simulink model "Sim5_MMC"  (R2021a)
settings: Solver=ode1  StartTime=0.0  StopTime=4  FixedStep=Time_Step  RelTol=1e-3
undefined symbols (not defined in the file): DiscIntNeverNeededParam, GRD00_Lg, GRD00_Rg, Time_Step, VSC01_id0
libraries: spsVoltageMeasurementLib x26, spsSeriesRLCBranchLib x24, Control_Lib x16, simulink x15, spsCurrentMeasurementLib x14, spsControlledCurrentSourceLib x12, spsControlledVoltageSourceLib x12, spsThreePhaseSourceLib x7, spsThreePhaseBreakerLib x6, spsThreePhaseVIMeasurementLib x5, spsLoadFlowBusLib x4, spsDCVoltageSourceLib x3
(part 1 of 5)
settings Model: Creator=fcolas  LastModifiedBy=fcolas
settings SolverCC: AlgebraicLoopSolver=TrustRegion
settings DebuggingCC: SFMachineParentedDataDiag=warning

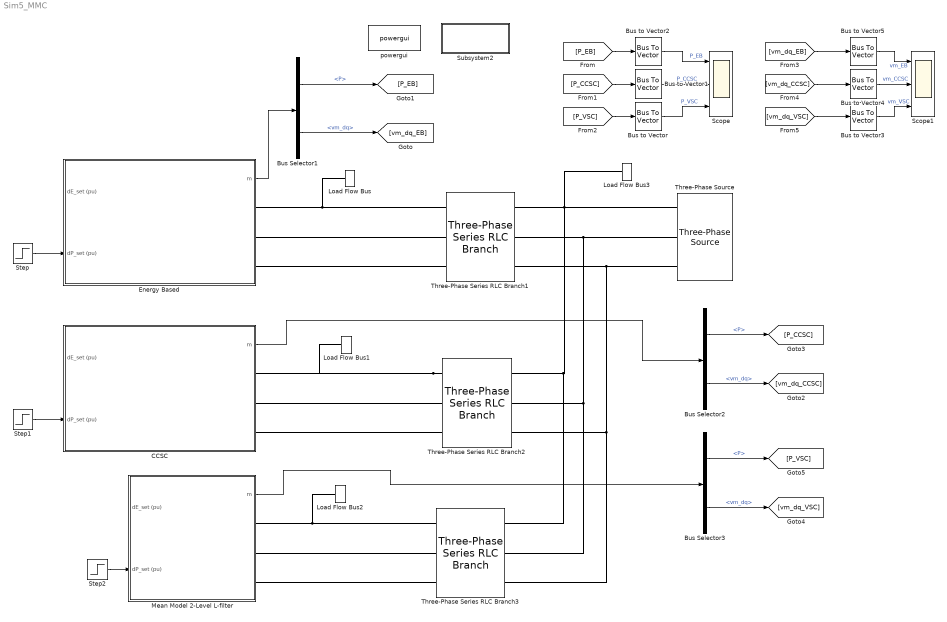
== system Sim5_MMC ==
  Bus Selector1 : BusSelector  OutputSignals=P,V.vm_dq
  Bus Selector2 : BusSelector  OutputSignals=P,V.vm_dq
  Bus Selector3 : BusSelector  OutputSignals=P,V.vm_dq
  Bus to Vector{,1..5} (6 alike) : BusToVector
  CCSC : Subsystem  mask(VSC){fn=50, Sn=1000e6, Pn=1000e6, Udcn=640e3, Time_Step=Time_Step, Un1=320e3, Un2=400e3, Rt_pu=0.005, Lt_pu=0.15, Lm_pu=500, Rm_pu=500, Larm_pu=0.18, Rarm_pu=0.005, nSM=0, Hc=40, Tr_PLL=100, Val_Freq_Support=off, R_percent=4, Rv=0.09, W_TVR=60, I_thresh_pu=1.2, DX_DR=5, Kp_Rvi_pu=0.676, I_max_pu=1.2, Tr_I_max=10, Diff_CC_fn=200, Diff_CC_zeta=1, fn_Wtot=5, zeta_Wtot=1, fn_Wdiff=3, zeta_Wdiff=1, Advanced=on, gainpopup=With Inertia, f_Inertia_Less=5, zeta_Inertia_Less=1, Param_Inertia=PI, H_GFo=5, zeta_GFo=1, LFpopup=PQ, P0=0.2, Q0=0, V0=1.0009, Theta0=0.57242}
      mask prompts: fn "Nominal Frequency (Hz)"; Sn "Nominal Apparent Power (VA)"; Pn "Nominal Power (W)"; Udcn "Nominal DC Voltage (V)"; Time_Step "Sample Time (s)"; Un1 "VSC side Nominal Ph-Ph Voltage (V)"; Un2 "Grid side Nominal Ph-Ph Voltage (V)"; Rt_pu "R (pu)"; Lt_pu "L (pu)"; Lm_pu "Rm (pu)"; Rm_pu "Lm (pu)"; Larm_pu "Arm Inductance (pu)"; Rarm_pu "Arm Resistance (pu)"; nSM "Sub-Modules number"; Hc "Hc (ms)"; Tr_PLL "Time response (ms)"; Val_Freq_Support "Frequency Support"; R_percent "Droop Gain (%)"; Rv "Damping Resistance (Rv)"; W_TVR "Dr filter"; I_thresh_pu "Current Threshold (pu)"; Kp_Rvi_pu "Kp_Rvi"; I_max_pu "I max (pu)"; Tr_I_max "Current Loop time response (ms)"; Diff_CC_fn "Bandwidth (Hz)"; Diff_CC_zeta "Damping"; fn_Wtot "Bandwidth (Hz)"; zeta_Wtot "Damping"; fn_Wdiff "Bandwidth (Hz)"; zeta_Wdiff "Damping"; gainpopup "Strategy"; f_Inertia_Less "Bandwidth (Hz)"; zeta_Inertia_Less "Damping"; H_GFo "Inertia H (s)"; zeta_GFo "Damping Ratio"; P0 "Initial Active Power (pu)"; Q0 "Initial Reactive Power (pu)"; V0 "Initial Voltage (pu)"; Theta0 "Initial Angle (°)"
      mask init:
      | % Update Name of LF bus for internal purpose
      |     %NameStr = [get_param(gcb,'Name')];% '_LF'];
      |     %set_param([gcb '/Load Flow Bus'],'ID',NameStr);    
      |     
      | % Base values
      |     fb = fn;
      |     Pb = Pn;
      |     cos_phi_n = Pn/Sn;
      |     Sb = Pb/cos_phi_n;
      |     Vn1 = Un1/sqrt(3);
      |     Vb1 = Vn1;
      |     Vn2 = Un2/sqrt(3);
      |     Vb2 = Vn2;
      |     Ib1 = Sb / 3*Vb1;
      |     Ib2 = Sb / (3*Vb2);
      |     wb = 2*pi*fb;
      |     Vdcb = Udcn;
      |     Idcb = Pb / Vdcb;
      |     Zb = (3*Vb1^2)/Sb;
      |     Lb = Zb/wb;
      |     Cb = 1/(Zb*wb);
      | 
      | % Average Model parameters
      |     Carm = 1/3*Pb/Vdcb^2*Hc/1000;
      |   
      | % PLL derivation of the parameters
      |     wn_PLL=5/Tr_PLL;
      |     zeta_PLL = 1;
      |     Kp_PLL_pu = 2*zeta_PLL*wn_PLL/wb;
      |     Ki_PLL_pu = wn_PLL^2/wb;
      |     
      | % Grid-Forming control tuning
      |     % Inertia Less
      |     wn_Inertia_Less = 2*pi*f_Inertia_Less;
      |     Ki_Inertia_Less = Lt_pu*wn_Inertia_Less^2/wb;
      |     Kp_Inertia_Less = 2*zeta_Inertia_Less*wn_Inertia_Less*Lt_pu/wb;
      |     
      |     % With Inertia
      |     Kc = 1/(Lt_pu+Larm_pu/2);
      |     kp_GFo = zeta_GFo*sqrt(2/(H_GFo*wb*Kc));
      |     kd = 2*H_GFo*kp_GFo*Kc*wb;
      |     
      | % Set the chosen strategy
      |     if (gainpopup == 1)
      |         Chosen_Strategy = 1;
      |     elseif (gainpopup == 2)
      |         if (Param_Inertia == 1)
      |             Chosen_Strategy = 2;
      |         elseif (Param_Inertia == 2)
      |             Chosen_Strategy = 3;
      |         end
      |     end
      | 
      | % Differential Current controller (CCSC)
      | 
      |     HL = 1/2*Larm_pu*Lb*Idcb^2/Pb; 
      |     Diff_CC_wn = 2*pi*Diff_CC_fn;
      |     Diff_CC_ki= 2*HL*Diff_CC_wn*Diff_CC_wn;
      |     Diff_CC_kp= (4*Diff_CC_zeta*Diff_CC_wn*HL)-(Rarm_pu);
      | 
      | %% Energy Sum W tot Per phase control design
      |     Hc_W    = 0.5*Carm*(Udcn^2)/Pn;    
      |     wn_Wtot     = 2*pi*fn_Wtot;
      |     Kp_Wtot_pu  = 2*zeta_Wtot*wn_Wtot*2*Hc_W;
      |     Ki_Wtot_pu  = wn_Wtot*wn_Wtot*2*Hc_W;
      | 
      | %% Control difference (balancing)  W diff Per phase control design  
      |     wn_Wdiff    = 2*pi*fn_Wdiff;
      |     Kp_Wdiff_pu = 2*zeta_Wdiff*wn_Wdiff*2*Hc_W;
      |     Ki_Wdiff_pu = wn_Wdiff*wn_Wdiff*2*Hc_W;
      |     
      | % Set the frequency droop gain
      |     R = R_percent / 100;
      | 
      | % Compute the delay compensation between control and power parts
      |     if (Time_Step == -1)
      |         Solver_Time_Step = 0;
      |     else
      |         Solver_Time_Step = Time_Step;
      |     end
      | 
      | % Compute Initial Voltage of VSC 
      | %   from steady-state output transformer model and Loadflow result
      |     
      |     %Initialize correctly the LoadFlow bus parameters connected to PCC
      |     VLF = V0;
      |     ThetaLF = Theta0;
      |     %if (LFpopup == 'PQ')
      |     %    VLF = 1;
      |     %    ThetaLF = 0;
      |     %elseif (LFpopup == 'PV')
      |     %%    VLF = V0;
      |     %    ThetaLF = 0;        
      |     %end
      |     %set_param([gcb '/Load Flow Bus'],'Vref',num2str(VLF),'Vangle',num2str(ThetaLF));
      |     
      |     R1_pu = Rt_pu/2+Rarm_pu/2;
      |     L1_pu = Lt_pu/2+Larm_pu/2;
      |     R2_pu = Rt_pu/2;
      |     L2_pu = Lt_pu/2;
      |     X1_pu = L1_pu;
      |     X2_pu = L2_pu;
      |     Xm_pu = Lm_pu;
      |     
      |     Zm_pu = 1/(1/Rm_pu+1/(1i*Xm_pu));
      | 
      |     S0=P0+1i*Q0;
      |     I2 = conj(S0)/(V0);
      | 
      |     Vm = (R2_pu+1i*X2_pu)*I2 + V0;
      |     Im = Vm/Zm_pu;
      | 
      |     I1 = I2 + Im;
      |     V1 = (R1_pu+1i*X1_pu) * I1 + Vm;
      | 
      |     Vvsc0 = abs(V1);
      |     Theta_vsc0 = angle(V1) * 180/pi+Theta0;
      |     
      |     Va0 = Vvsc0*sqrt(2)*Vb1*sin(Theta_vsc0*pi/180);
      |     Vb0 = Vvsc0*sqrt(2)*Vb1*sin(Theta_vsc0*pi/180-2*pi/3);
      |     Vc0 = Vvsc0*sqrt(2)*Vb1*sin(Theta_vsc0*pi/180+2*pi/3);
      |     
      | % Generate string to display LF results on Mask
      |     %str_tmp = fprintf("Vvsc0 = %d, Theta_vsc0 = %d°",Vvsc0,Theta_vsc0);
      |     mo = get_param(gcb,'MaskObject');
      |     mo.getDialogControl('LF_vsc_str').Prompt = ['V0 = ', num2str(Vvsc0),' pu, Angle = ', num2str(Theta_vsc0),'°'];
      |     mo.getDialogControl('LF_pcc_str').Prompt = ['V0 = ', num2str(V0),' pu, Angle = ', num2str(Theta0),'°'];
      |     mo.getDialogControl('LF_pcc_Power_str').Prompt = ['P0 = ', num2str(P0),' pu, Q0 = ', num2str(Q0),' pu'];
      |     %set_param([gcb],'LF_str',str_tmp);
      settings: OpenFcn=|
      | NameStr = get_param(gcb,'Name');
      | open_system(gcbh, 'Mask');
      | 
      | h2AllOpenDlgs = DAStudio.ToolRoot.getOpenDialogs;
      | 
      | for i=1:length(h2AllOpenDlgs)
      |     try
      |          %disp(h2AllOpenDlgs(i).getSource.getBlock.Name);
      |         Dialog_block_name = h2AllOpenDlgs(i).getSource.getBlock.Name;
      |          %strcmp(Dialog_block_name, NameStr),
      |         if (strcmp(h2AllOpenDlgs(i).getSource.getBlock.Name, NameStr))
      |             iPos = h2AllOpenDlgs(i).position;
      |             h2AllOpenDlgs(i).position = [iPos(1)   iPos(2)   iPos(3)*1.4   iPos(4)];
      |         end
      |     end
      | end
      mask Callback Advanced:
      | % Get the mask parameter values. This is a cell
      | %   array of character vectors.
      | maskStr = get_param(gcb,'Advanced');
      | p=Simulink.Mask.get(gcb);
      | 
      | % The pop-up menu is the first mask parameter.
      | %   Check the value selected in the pop-up
      | if strcmp(maskStr,'on'),
      | 
      |     % Set the visibility of both parameters on when
      |     %   User-defined is selected in the pop-up.
      |     p.getDialogControl('TVR').Visible='on';
      |     p.getDialogControl('TVI').Visible='on';
      |     %p.getDialogControl('LC_Filter').Visible='on';
      |     p.getDialogControl('Current_Sat').Visible='on';
      |     p.getDialogControl('MMC_Control').Visible='on';
      |     %p.getDialogControl('Param_Strat_3').Visible='off';
      | 
      | 
      | else
      | 
      |     % Set the visibility of both parameters on when
      |     %   User-defined is selected in the pop-up.
      |     p.getDialogControl('TVR').Visible='off';
      |     p.getDialogControl('TVI').Visible='off';
      |     %p.getDialogControl('LC_Filter').Visible='off';
      |     p.getDialogControl('Current_Sat').Visible='off';
      |     p.getDialogControl('MMC_Control').Visible='off';
      |     %p.getDialogControl('Param_Strat_3').Visible='off';
      | 
      | end
      mask TypeOptions gainpopup: Inertia Less | With Inertia
      mask Callback gainpopup:
      | % Get the mask parameter values. This is a cell
      | %   array of character vectors.
      | maskStr = get_param(gcb,'gainpopup');
      | p=Simulink.Mask.get(gcb);
      | 
      | % The pop-up menu is the first mask parameter.
      | %   Check the value selected in the pop-up
      | if strcmp(maskStr,'Inertia Less'),
      | 
      |     % Set the visibility of both parameters on when
      |     %   User-defined is selected in the pop-up.
      |     p.getDialogControl('No_Inertia').Visible='on';
      |     p.getDialogControl('Inertia').Visible='off';
      |     %p.getDialogControl('Param_Strat_3').Visible='off';
      | 
      | 
      | elseif strcmp(maskStr,'With Inertia'),
      | 
      |     % Set the visibility of both parameters on when
      |     %   User-defined is selected in the pop-up.
      |     p.getDialogControl('No_Inertia').Visible='off';
      |     p.getDialogControl('Inertia').Visible='on';
      |     %p.getDialogControl('Param_Strat_3').Visible='off';
      | 
      | 
      |     % Turn off the visibility of the Value field
      |     %   when User-defined is not selected.
      | 
      | else
      | 
      |     % Set the visibility of both parameters on when
      |     %   User-defined is selected in the pop-up.
      |     p.getDialogControl('No_Inertia').Visible='off';
      |     p.getDialogControl('Inertia').Visible='off';
      |     %p.getDialogControl('Param_Strat_3').Visible='off';
      | 
      | end
      mask TypeOptions Param_Inertia: VSM | PI
      mask TypeOptions LFpopup: Swing | PQ | PV
      mask Callback LFpopup:
      | % Get the mask parameter values. This is a cell
      | %   array of character vectors.
      | maskStr = get_param(gcb,'LFpopup');
      | p=Simulink.Mask.get(gcb);
      | 
      | % The pop-up menu is the first mask parameter.
      | %   Check the value selected in the pop-up
      | if strcmp(maskStr,'Swing'),
      | 
      |     % Set the visibility of both parameters on when
      |     %   User-defined is selected in the pop-up.
      |     p.getParameter('P0').Visible='off';
      |     p.getParameter('Q0').Visible='off';
      |     p.getParameter('V0').Visible='on';
      |     p.getParameter('Theta0').Visible='on';
      |     set_param([gcb '/Source_For_LF'],'BusType','swing');
      | 
      | elseif strcmp(maskStr,'PQ'),
      | 
      |     % Set the visibility of both parameters on when
      |     %   User-defined is selected in the pop-up.
      |     p.getParameter('P0').Visible='on';
      |     p.getParameter('Q0').Visible='on';
      |     p.getParameter('V0').Visible='off';
      |     p.getParameter('Theta0').Visible='off';
      |     set_param([gcb '/Source_For_LF'],'BusType','PQ');
      | 
      |     % Turn off the visibility of the Value field
      |     %   when User-defined is not selected.
      | else
      | 
      |     % Set the visibility of both parameters on when
      |     %   User-defined is selected in the pop-up.
      |     p.getParameter('P0').Visible='on';
      |     p.getParameter('Q0').Visible='off';
      |     p.getParameter('V0').Visible='on';
      |     p.getParameter('Theta0').Visible='off';
      |     set_param([gcb '/Source_For_LF'],'BusType','PV');
      | 
      | end
      mask DialogControl Nominal_Param Prompt: Nominal Value
      mask DialogControl Container20 Prompt: Passive Components
      mask DialogControl Container21 Prompt: Output Transformer
      mask DialogControl Container22 Prompt: Sub-Modules & Arm
      mask DialogControl Control_Param Prompt: Control Parameter
      mask DialogControl Container13 Prompt: PLL
      mask DialogControl Container14 Prompt: Frequency Support
      mask DialogControl TVR Prompt: Transient Virtual Resistor
      mask DialogControl TVI Prompt: Virtual Impedance
      mask DialogControl Current_Sat Prompt: Current Limitation
      mask DialogControl MMC_Control Prompt: MMC Controller
      mask DialogControl Container27 Prompt: Differential Current Controller
      mask DialogControl Container26 Prompt: Wtot Controller
      mask DialogControl Container28 Prompt: Wdiff Controller
      mask DialogControl Container18 Prompt: Control Strategy
      mask DialogControl LF_Param Prompt: Loadflow
      mask DialogControl Control4 Prompt: Initial Operating Point
      mask DialogControl Container24 Prompt: VSC side
      mask DialogControl LF_vsc_str Prompt: V0 = 1.0039 pu, Angle = 3.3291°
      mask DialogControl Container25 Prompt: PCC
      mask DialogControl LF_pcc_str Prompt: V0 = 1.0009 pu, Angle = 0.57242°
      mask DialogControl LF_pcc_Power_str Prompt: P0 = 0.2 pu, Q0 = 0 pu
      mask DialogControl UpdateLoadflow Prompt: Update Loadflow
      mask DialogControl UpdateLoadflow Callback: LoadFlow_VSC
      mask Display:
      | % Q1
      | x1=-0.07;
      | y1=+0.03;
      | plot([0.4 0.4]+x1,[0.90,0.80]+y1)
      | plot([0.4 0.33]+x1,[0.80 0.74]+y1)
      | plot([0.33 0.33]+x1,[0.78 0.66]+y1)
      | plot([0.33 0.4]+x1,[0.70 0.64]+y1)
      | plot([0.4 0.4]+x1,[0.64 0.55]+y1)
      | plot([0.38 0.40 0.35]+x1,[0.68 0.64 0.64]+y1)
      | plot([0.30 0.30]+x1,[0.74 0.7]+y1)
      | plot([0.29 0.27]+x1,[0.72 0.72]+y1)
      | % Q2
      | y1=y1-0.51;
      | plot([0.4 0.4]+x1,[0.90,0.80]+y1)
      | plot([0.4 0.33]+x1,[0.80 0.74]+y1)
      | plot([0.33 0.33]+x1,[0.78 0.66]+y1)
      | plot([0.33 0.4]+x1,[0.70 0.64]+y1)
      | plot([0.4 0.4]+x1,[0.64 0.55]+y1)
      | plot([0.39 0.40 0.35]+x1,[0.68 0.64 0.64]+y1)
      | plot([0.30 0.30]+x1,[0.75 0.7]+y1)
      | plot([0.29 0.27]+x1,[0.72 0.72]+y1)
      | % Q3
      | y1=y1+0.51;
      | x1=x1+0.22+0.1;
      | plot([0.4 0.4]+x1,[0.90,0.80]+y1)
      | plot([0.4 0.33]+x1,[0.80 0.74]+y1)
      | plot([0.33 0.33]+x1,[0.78 0.66]+y1)
      | plot([0.33 0.4]+x1,[0.70 0.64]+y1)
      | plot([0.4 0.4]+x1,[0.64 0.55]+y1)
      | plot([0.39 0.41 0.34]+x1,[0.68 0.64 0.64]+y1)
      | plot([0.30 0.30]+x1,[0.75 0.7]+y1)
      | plot([0.29 0.27]+x1,[0.72 0.72]+y1)
      | % Q4
      | y1=y1-0.51;
      | x1=x1;
      | plot([0.4 0.4]+x1,[0.90,0.80]+y1)
      | plot([0.4 0.33]+x1,[0.80 0.74]+y1)
      | plot([0.33 0.33]+x1,[0.78 0.66]+y1)
      | plot([0.33 0.4]+x1,[0.70 0.64]+y1)
      | plot([0.4 0.4]+x1,[0.64 0.55]+y1)
      | plot([0.39 0.41 0.34]+x1,[0.68 0.64 0.64]+y1)
      | plot([0.30 0.30]+x1,[0.75 0.7]+y1)
      | plot([0.29 0.26]+x1,[0.72 0.72]+y1)
      | %
      | x1=-0.05;
      | y1=+0.03;
      | plot([0.90 0.40]+x1,[0.9 0.9]+y1)
      | plot([0.90 0.40]+x1,[0.04 0.04]+y1)
      | %
      | 
      | plot([0.69 0.42]+x1,[0.4 0.4]+y1)
      | plot([0.38 0.22]+x1,[0.52 0.52]+y1)
      | plot([0.22 0.22]+x1,[0.52 0.54]+y1)
      | plot([0.22 0.22]+x1,[0.56 0.58]+y1)
      | plot([0.22 0.22]+x1,[0.60 0.63]+y1)
      | %
      | plot([0.35 0.22]+x1,[0.4 0.4]+y1)
      | plot([0.22 0.22]+x1,[0.4 0.37]+y1)
      | plot([0.22 0.22]+x1,[0.4 0.37]+y1)
      | plot([0.22 0.22]+x1,[0.35 0.32]+y1)
      | plot([0.22 0.22]+x1,[0.30 0.27]+y1)
      | %
      | plot([0.38 0.38]+x1,[ 0.55 0.38]+y1)
      | plot([0.7 0.7]+x1,[0.55 0.3]+y1)
      | %
      | % D1
      | x1=-0.07;
      | y1=+0.03;
      | plot([0.4 0.45]+x1,[0.84,0.84]+y1)
      | plot([0.45 0.45]+x1,[0.84,0.75]+y1)
      | plot([0.45 0.41]+x1,[0.75,0.72]+y1)
      | plot([0.45 0.48]+x1,[0.75,0.72]+y1)
      | plot([0.41 0.48]+x1,[0.72,0.72]+y1)
      | plot([0.45 0.45]+x1,[0.72,0.6]+y1)
      | plot([0.4 0.45]+x1,[0.6,0.6]+y1)
      | % D2
      | x1=x1+0.22+0.1;
      | plot([0.4 0.45]+x1,[0.84,0.84]+y1)
      | plot([0.45 0.45]+x1,[0.84,0.75]+y1)
      | plot([0.45 0.43]+x1,[0.75,0.72]+y1)
      | plot([0.45 0.48]+x1,[0.75,0.72]+y1)
      | %
      | plot([0.43 0.48]+x1,[0.72,0.72]+y1)
      | plot([0.45 0.45]+x1,[0.72,0.6]+y1)
      | plot([0.4 0.45]+x1,[0.6,0.6]+y1)
      | % D3
      | x1=x1-0.22-0.1;
      | y1=y1-0.5;
      | plot([0.4 0.45]+x1,[0.84,0.84]+y1)
      | plot([0.45 0.45]+x1,[0.84,0.75]+y1)
      | plot([0.45 0.41]+x1,[0.75,0.72]+y1)
      | plot([0.45 0.48]+x1,[0.75,0.72]+y1)
      | plot([0.41 0.48]+x1,[0.72,0.72]+y1)
      | plot([0.45 0.45]+x1,[0.72,0.6]+y1)
      | plot([0.4 0.45]+x1,[0.6,0.6]+y1)
      | % D4
      | x1=x1+0.22+0.1;
      | plot([0.4 0.45]+x1,[0.84,0.84]+y1)
      | plot([0.45 0.45]+x1,[0.84,0.75]+y1)
      | plot([0.45 0.43]+x1,[0.75,0.72]+y1)
      | plot([0.45 0.48]+x1,[0.75,0.72]+y1)
      | plot([0.43 0.48]+x1,[0.72,0.72]+y1)
      | plot([0.45 0.45]+x1,[0.72,0.6]+y1)
      | plot([0.40 0.45]+x1,[0.6,0.6]+y1)
      | disp('MMC GFo');
      | port_label('input',1,'dE_set (pu)');
      | port_label('input',2,'dP_set (pu)');
      | port_label('output',1,'m');
      | port_label('rconn',1,'A');
      | port_label('rconn',2,'B');
      | port_label('rconn',3,'C');
  Energy Based : Subsystem  mask(VSC){fn=50, Sn=1000e6, Pn=1000e6, Udcn=640e3, Time_Step=Time_Step, Un1=320e3, Un2=400e3, Rt_pu=0.005, Lt_pu=0.15, Lm_pu=500, Rm_pu=500, Larm_pu=0.18, Rarm_pu=0.005, nSM=0, Hc=40, Tr_PLL=100, Val_Freq_Support=off, R_percent=4, Rv=0.09, W_TVR=60, I_thresh_pu=1.2, DX_DR=5, Kp_Rvi_pu=0.676, I_max_pu=1.2, Tr_I_max=10, Diff_CC_fn=200, Diff_CC_zeta=1, fn_Wtot=5, zeta_Wtot=1, fn_Wdiff=3, zeta_Wdiff=1, Advanced=on, gainpopup=With Inertia, f_Inertia_Less=5, zeta_Inertia_Less=1, Param_Inertia=PI, H_GFo=5, zeta_GFo=0.7, LFpopup=PQ, P0=0.2, Q0=0, V0=1.0009, Theta0=0.57242}
      mask prompts: fn "Nominal Frequency (Hz)"; Sn "Nominal Apparent Power (VA)"; Pn "Nominal Power (W)"; Udcn "Nominal DC Voltage (V)"; Time_Step "Sample Time (s)"; Un1 "VSC side Nominal Ph-Ph Voltage (V)"; Un2 "Grid side Nominal Ph-Ph Voltage (V)"; Rt_pu "R (pu)"; Lt_pu "L (pu)"; Lm_pu "Rm (pu)"; Rm_pu "Lm (pu)"; Larm_pu "Arm Inductance (pu)"; Rarm_pu "Arm Resistance (pu)"; nSM "Sub-Modules number"; Hc "Hc (ms)"; Tr_PLL "Time response (ms)"; Val_Freq_Support "Frequency Support"; R_percent "Droop Gain (%)"; Rv "Damping Resistance (Rv)"; W_TVR "Dr filter"; I_thresh_pu "Current Threshold (pu)"; Kp_Rvi_pu "Kp_Rvi"; I_max_pu "I max (pu)"; Tr_I_max "Current Loop time response (ms)"; Diff_CC_fn "Bandwidth (Hz)"; Diff_CC_zeta "Damping"; fn_Wtot "Bandwidth (Hz)"; zeta_Wtot "Damping"; fn_Wdiff "Bandwidth (Hz)"; zeta_Wdiff "Damping"; gainpopup "Strategy"; f_Inertia_Less "Bandwidth (Hz)"; zeta_Inertia_Less "Damping"; H_GFo "Inertia H (s)"; zeta_GFo "Damping Ratio"; P0 "Initial Active Power (pu)"; Q0 "Initial Reactive Power (pu)"; V0 "Initial Voltage (pu)"; Theta0 "Initial Angle (°)"
      mask init: same as Sim5_MMC/CCSC
      settings: OpenFcn=|
      | NameStr = get_param(gcb,'Name');
      | open_system(gcbh, 'Mask');
      | 
      | h2AllOpenDlgs = DAStudio.ToolRoot.getOpenDialogs;
      | 
      | for i=1:length(h2AllOpenDlgs)
      |     try
      |          %disp(h2AllOpenDlgs(i).getSource.getBlock.Name);
      |         Dialog_block_name = h2AllOpenDlgs(i).getSource.getBlock.Name;
      |          %strcmp(Dialog_block_name, NameStr),
      |         if (strcmp(h2AllOpenDlgs(i).getSource.getBlock.Name, NameStr))
      |             iPos = h2AllOpenDlgs(i).position;
      |             h2AllOpenDlgs(i).position = [iPos(1)   iPos(2)   iPos(3)*1.4   iPos(4)];
      |         end
      |     end
      | end
      mask Callback Advanced:
      | % Get the mask parameter values. This is a cell
      | %   array of character vectors.
      | maskStr = get_param(gcb,'Advanced');
      | p=Simulink.Mask.get(gcb);
      | 
      | % The pop-up menu is the first mask parameter.
      | %   Check the value selected in the pop-up
      | if strcmp(maskStr,'on'),
      | 
      |     % Set the visibility of both parameters on when
      |     %   User-defined is selected in the pop-up.
      |     p.getDialogControl('TVR').Visible='on';
      |     p.getDialogControl('TVI').Visible='on';
      |     %p.getDialogControl('LC_Filter').Visible='on';
      |     p.getDialogControl('Current_Sat').Visible='on';
      |     p.getDialogControl('MMC_Control').Visible='on';
      |     %p.getDialogControl('Param_Strat_3').Visible='off';
      | 
      | 
      | else
      | 
      |     % Set the visibility of both parameters on when
      |     %   User-defined is selected in the pop-up.
      |     p.getDialogControl('TVR').Visible='off';
      |     p.getDialogControl('TVI').Visible='off';
      |     %p.getDialogControl('LC_Filter').Visible='off';
      |     p.getDialogControl('Current_Sat').Visible='off';
      |     p.getDialogControl('MMC_Control').Visible='off';
      |     %p.getDialogControl('Param_Strat_3').Visible='off';
      | 
      | end
      mask TypeOptions gainpopup: Inertia Less | With Inertia
      mask Callback gainpopup:
      | % Get the mask parameter values. This is a cell
      | %   array of character vectors.
      | maskStr = get_param(gcb,'gainpopup');
      | p=Simulink.Mask.get(gcb);
      | 
      | % The pop-up menu is the first mask parameter.
      | %   Check the value selected in the pop-up
      | if strcmp(maskStr,'Inertia Less'),
      | 
      |     % Set the visibility of both parameters on when
      |     %   User-defined is selected in the pop-up.
      |     p.getDialogControl('No_Inertia').Visible='on';
      |     p.getDialogControl('Inertia').Visible='off';
      |     %p.getDialogControl('Param_Strat_3').Visible='off';
      | 
      | 
      | elseif strcmp(maskStr,'With Inertia'),
      | 
      |     % Set the visibility of both parameters on when
      |     %   User-defined is selected in the pop-up.
      |     p.getDialogControl('No_Inertia').Visible='off';
      |     p.getDialogControl('Inertia').Visible='on';
      |     %p.getDialogControl('Param_Strat_3').Visible='off';
      | 
      | 
      |     % Turn off the visibility of the Value field
      |     %   when User-defined is not selected.
      | 
      | else
      | 
      |     % Set the visibility of both parameters on when
      |     %   User-defined is selected in the pop-up.
      |     p.getDialogControl('No_Inertia').Visible='off';
      |     p.getDialogControl('Inertia').Visible='off';
      |     %p.getDialogControl('Param_Strat_3').Visible='off';
      | 
      | end
      mask TypeOptions Param_Inertia: VSM | PI
      mask TypeOptions LFpopup: Swing | PQ | PV
      mask Callback LFpopup:
      | % Get the mask parameter values. This is a cell
      | %   array of character vectors.
      | maskStr = get_param(gcb,'LFpopup');
      | p=Simulink.Mask.get(gcb);
      | 
      | % The pop-up menu is the first mask parameter.
      | %   Check the value selected in the pop-up
      | if strcmp(maskStr,'Swing'),
      | 
      |     % Set the visibility of both parameters on when
      |     %   User-defined is selected in the pop-up.
      |     p.getParameter('P0').Visible='off';
      |     p.getParameter('Q0').Visible='off';
      |     p.getParameter('V0').Visible='on';
      |     p.getParameter('Theta0').Visible='on';
      |     set_param([gcb '/Source_For_LF'],'BusType','swing');
      | 
      | elseif strcmp(maskStr,'PQ'),
      | 
      |     % Set the visibility of both parameters on when
      |     %   User-defined is selected in the pop-up.
      |     p.getParameter('P0').Visible='on';
      |     p.getParameter('Q0').Visible='on';
      |     p.getParameter('V0').Visible='off';
      |     p.getParameter('Theta0').Visible='off';
      |     set_param([gcb '/Source_For_LF'],'BusType','PQ');
      | 
      |     % Turn off the visibility of the Value field
      |     %   when User-defined is not selected.
      | else
      | 
      |     % Set the visibility of both parameters on when
      |     %   User-defined is selected in the pop-up.
      |     p.getParameter('P0').Visible='on';
      |     p.getParameter('Q0').Visible='off';
      |     p.getParameter('V0').Visible='on';
      |     p.getParameter('Theta0').Visible='off';
      |     set_param([gcb '/Source_For_LF'],'BusType','PV');
      | 
      | end
      mask DialogControl Nominal_Param Prompt: Nominal Value
      mask DialogControl Container20 Prompt: Passive Components
      mask DialogControl Container21 Prompt: Output Transformer
      mask DialogControl Container22 Prompt: Sub-Modules & Arm
      mask DialogControl Control_Param Prompt: Control Parameter
      mask DialogControl Container13 Prompt: PLL
      mask DialogControl Container14 Prompt: Frequency Support
      mask DialogControl TVR Prompt: Transient Virtual Resistor
      mask DialogControl TVI Prompt: Virtual Impedance
      mask DialogControl Current_Sat Prompt: Current Limitation
      mask DialogControl MMC_Control Prompt: MMC Controller
      mask DialogControl Container27 Prompt: Differential Current Controller
      mask DialogControl Container26 Prompt: Wtot Controller
      mask DialogControl Container28 Prompt: Wdiff Controller
      mask DialogControl Container18 Prompt: Control Strategy
      mask DialogControl LF_Param Prompt: Loadflow
      mask DialogControl Control4 Prompt: Initial Operating Point
      mask DialogControl Container24 Prompt: VSC side
      mask DialogControl LF_vsc_str Prompt: V0 = 1.0039 pu, Angle = 3.3291°
      mask DialogControl Container25 Prompt: PCC
      mask DialogControl LF_pcc_str Prompt: V0 = 1.0009 pu, Angle = 0.57242°
      mask DialogControl LF_pcc_Power_str Prompt: P0 = 0.2 pu, Q0 = 0 pu
      mask DialogControl UpdateLoadflow Prompt: Update Loadflow
      mask DialogControl UpdateLoadflow Callback: LoadFlow_VSC
      mask Display:
      | % Q1
      | x1=-0.07;
      | y1=+0.03;
      | plot([0.4 0.4]+x1,[0.90,0.80]+y1)
      | plot([0.4 0.33]+x1,[0.80 0.74]+y1)
      | plot([0.33 0.33]+x1,[0.78 0.66]+y1)
      | plot([0.33 0.4]+x1,[0.70 0.64]+y1)
      | plot([0.4 0.4]+x1,[0.64 0.55]+y1)
      | plot([0.38 0.40 0.35]+x1,[0.68 0.64 0.64]+y1)
      | plot([0.30 0.30]+x1,[0.74 0.7]+y1)
      | plot([0.29 0.27]+x1,[0.72 0.72]+y1)
      | % Q2
      | y1=y1-0.51;
      | plot([0.4 0.4]+x1,[0.90,0.80]+y1)
      | plot([0.4 0.33]+x1,[0.80 0.74]+y1)
      | plot([0.33 0.33]+x1,[0.78 0.66]+y1)
      | plot([0.33 0.4]+x1,[0.70 0.64]+y1)
      | plot([0.4 0.4]+x1,[0.64 0.55]+y1)
      | plot([0.39 0.40 0.35]+x1,[0.68 0.64 0.64]+y1)
      | plot([0.30 0.30]+x1,[0.75 0.7]+y1)
      | plot([0.29 0.27]+x1,[0.72 0.72]+y1)
      | % Q3
      | y1=y1+0.51;
      | x1=x1+0.22+0.1;
      | plot([0.4 0.4]+x1,[0.90,0.80]+y1)
      | plot([0.4 0.33]+x1,[0.80 0.74]+y1)
      | plot([0.33 0.33]+x1,[0.78 0.66]+y1)
      | plot([0.33 0.4]+x1,[0.70 0.64]+y1)
      | plot([0.4 0.4]+x1,[0.64 0.55]+y1)
      | plot([0.39 0.41 0.34]+x1,[0.68 0.64 0.64]+y1)
      | plot([0.30 0.30]+x1,[0.75 0.7]+y1)
      | plot([0.29 0.27]+x1,[0.72 0.72]+y1)
      | % Q4
      | y1=y1-0.51;
      | x1=x1;
      | plot([0.4 0.4]+x1,[0.90,0.80]+y1)
      | plot([0.4 0.33]+x1,[0.80 0.74]+y1)
      | plot([0.33 0.33]+x1,[0.78 0.66]+y1)
      | plot([0.33 0.4]+x1,[0.70 0.64]+y1)
      | plot([0.4 0.4]+x1,[0.64 0.55]+y1)
      | plot([0.39 0.41 0.34]+x1,[0.68 0.64 0.64]+y1)
      | plot([0.30 0.30]+x1,[0.75 0.7]+y1)
      | plot([0.29 0.26]+x1,[0.72 0.72]+y1)
      | %
      | x1=-0.05;
      | y1=+0.03;
      | plot([0.90 0.40]+x1,[0.9 0.9]+y1)
      | plot([0.90 0.40]+x1,[0.04 0.04]+y1)
      | %
      | 
      | plot([0.69 0.42]+x1,[0.4 0.4]+y1)
      | plot([0.38 0.22]+x1,[0.52 0.52]+y1)
      | plot([0.22 0.22]+x1,[0.52 0.54]+y1)
      | plot([0.22 0.22]+x1,[0.56 0.58]+y1)
      | plot([0.22 0.22]+x1,[0.60 0.63]+y1)
      | %
      | plot([0.35 0.22]+x1,[0.4 0.4]+y1)
      | plot([0.22 0.22]+x1,[0.4 0.37]+y1)
      | plot([0.22 0.22]+x1,[0.4 0.37]+y1)
      | plot([0.22 0.22]+x1,[0.35 0.32]+y1)
      | plot([0.22 0.22]+x1,[0.30 0.27]+y1)
      | %
      | plot([0.38 0.38]+x1,[ 0.55 0.38]+y1)
      | plot([0.7 0.7]+x1,[0.55 0.3]+y1)
      | %
      | % D1
      | x1=-0.07;
      | y1=+0.03;
      | plot([0.4 0.45]+x1,[0.84,0.84]+y1)
      | plot([0.45 0.45]+x1,[0.84,0.75]+y1)
      | plot([0.45 0.41]+x1,[0.75,0.72]+y1)
      | plot([0.45 0.48]+x1,[0.75,0.72]+y1)
      | plot([0.41 0.48]+x1,[0.72,0.72]+y1)
      | plot([0.45 0.45]+x1,[0.72,0.6]+y1)
      | plot([0.4 0.45]+x1,[0.6,0.6]+y1)
      | % D2
      | x1=x1+0.22+0.1;
      | plot([0.4 0.45]+x1,[0.84,0.84]+y1)
      | plot([0.45 0.45]+x1,[0.84,0.75]+y1)
      | plot([0.45 0.43]+x1,[0.75,0.72]+y1)
      | plot([0.45 0.48]+x1,[0.75,0.72]+y1)
      | %
      | plot([0.43 0.48]+x1,[0.72,0.72]+y1)
      | plot([0.45 0.45]+x1,[0.72,0.6]+y1)
      | plot([0.4 0.45]+x1,[0.6,0.6]+y1)
      | % D3
      | x1=x1-0.22-0.1;
      | y1=y1-0.5;
      | plot([0.4 0.45]+x1,[0.84,0.84]+y1)
      | plot([0.45 0.45]+x1,[0.84,0.75]+y1)
      | plot([0.45 0.41]+x1,[0.75,0.72]+y1)
      | plot([0.45 0.48]+x1,[0.75,0.72]+y1)
      | plot([0.41 0.48]+x1,[0.72,0.72]+y1)
      | plot([0.45 0.45]+x1,[0.72,0.6]+y1)
      | plot([0.4 0.45]+x1,[0.6,0.6]+y1)
      | % D4
      | x1=x1+0.22+0.1;
      | plot([0.4 0.45]+x1,[0.84,0.84]+y1)
      | plot([0.45 0.45]+x1,[0.84,0.75]+y1)
      | plot([0.45 0.43]+x1,[0.75,0.72]+y1)
      | plot([0.45 0.48]+x1,[0.75,0.72]+y1)
      | plot([0.43 0.48]+x1,[0.72,0.72]+y1)
      | plot([0.45 0.45]+x1,[0.72,0.6]+y1)
      | plot([0.40 0.45]+x1,[0.6,0.6]+y1)
      | disp('MMC GFo');
      | port_label('input',1,'dE_set (pu)');
      | port_label('input',2,'dP_set (pu)');
      | port_label('output',1,'m');
      | port_label('rconn',1,'A');
      | port_label('rconn',2,'B');
      | port_label('rconn',3,'C');
  Load Flow Bus : spsLoadFlowBusLib/Load Flow Bus  LConnTagsString=a  Phases=single  Connectors=on one side  ID=BUS_1  Vbase=400e3  Vref=1  Vangle=0  VLF=1.001  VLFb=1  VLFc=1  angleLF=0.5724  angleLFb=0  angleLFc=0
      settings: SourceProductBaseCode=PS
  Load Flow Bus1 : spsLoadFlowBusLib/Load Flow Bus  LConnTagsString=a  Phases=single  Connectors=on one side  ID=BUS_2  Vbase=400e3  Vref=1  Vangle=0  VLF=1.001  VLFb=1  VLFc=1  angleLF=0.5724  angleLFb=0  angleLFc=0
      settings: SourceProductBaseCode=PS
  Load Flow Bus2 : spsLoadFlowBusLib/Load Flow Bus  LConnTagsString=a  Phases=single  Connectors=on one side  ID=BUS_3  Vbase=400e3  Vref=1  Vangle=0  VLF=1.001  VLFb=1  VLFc=1  angleLF=0.5724  angleLFb=0  angleLFc=0
      settings: SourceProductBaseCode=PS
  Load Flow Bus3 : spsLoadFlowBusLib/Load Flow Bus  LConnTagsString=a  Phases=single  Connectors=on one side  ID=BUS_0  Vbase=400e3  Vref=1  Vangle=0  VLF=1  VLFb=1  VLFc=1  angleLF=0  angleLFb=0  angleLFc=0
      settings: SourceProductBaseCode=PS
  Mean Model 2-Level L-filter : Subsystem  mask(VSC){fn=50, Sn=1000e6, Pn=1000e6, Udcn=640e3, Time_Step=Time_Step, Un1=320e3, Un2=400e3, Rt_pu=0.005+0.005/2, Lt_pu=0.15+0.18/2, Lm_pu=500, Rm_pu=500, Tr_PLL=100, Val_Freq_Support=off, R_percent=4, Rv=0.09, W_TVR=60, I_max_VI_pu=1.2, DX_DR=5, Val_Mod_H=off, I_max_pu=1.2, Tr_I_max=10, Advanced=on, gainpopup=With Inertia, f_Inertia_Less=5, zeta_Inertia_Less=1, Param_Inertia=PI, H_GFo=5, zeta_GFo=0.7, LFpopup=PQ, P0=0.2, Q0=4.3368e-19, V0=1.0009, Theta0=0.57242}
      mask prompts: fn "Nominal Frequency (Hz)"; Sn "Nominal Apparent Power (VA)"; Pn "Nominal Power (W)"; Udcn "Nominal DC Voltage (V)"; Time_Step "Sample Time (s)"; Un1 "VSC side Nominal Ph-Ph Voltage (V)"; Un2 "Grid side Nominal Ph-Ph Voltage (V)"; Rt_pu "R (pu)"; Lt_pu "L (pu)"; Lm_pu "Rm (pu)"; Rm_pu "Lm (pu)"; Tr_PLL "Time response (ms)"; Val_Freq_Support "Frequency Support"; R_percent "Droop Gain (%)"; Rv "Damping Resistance (Rv)"; W_TVR "Dr filter"; I_max_VI_pu "Current Threshold (pu)"; Val_Mod_H "Inertia Modulation"; I_max_pu "I max (pu)"; Tr_I_max "Current Loop time response (ms)"; gainpopup "Strategy"; f_Inertia_Less "Bandwidth (Hz)"; zeta_Inertia_Less "Damping"; H_GFo "Inertia H (s)"; zeta_GFo "Damping Ratio"; P0 "Initial Active Power (pu)"; Q0 "Initial Reactive Power (pu)"; V0 "Initial Voltage (pu)"; Theta0 "Initial Angle (°)"
      mask init:
      | % Update Name of LF bus for internal purpose
      |     %NameStr = [get_param(gcb,'Name')];% '_LF'];
      |     %set_param([gcb '/Load Flow Bus'],'ID',NameStr);    
      |     
      | % Base values
      |     fb = fn;
      |     Pb = Pn;
      |     cos_phi_n = Pn/Sn;
      |     Sb = Pb/cos_phi_n;
      |     Vn1 = Un1/sqrt(3);
      |     Vb1 = Vn1;
      |     Vn2 = Un2/sqrt(3);
      |     Vb2 = Vn2;
      |     Ib1 = Sb / 3*Vb1;
      |     Ib2 = Sb / (3*Vb2);
      |     wb = 2*pi*fb;
      |   
      | % PLL derivation of the parameters
      |     wn_PLL=5/Tr_PLL;
      |     zeta_PLL = 1;
      |     Kp_PLL_pu = 2*zeta_PLL*wn_PLL/wb;
      |     Ki_PLL_pu = wn_PLL^2/wb;
      |     
      | % Grid-Forming control tuning
      |     % Inertia Less
      |     wn_Inertia_Less = 2*pi*f_Inertia_Less;
      |     Ki_Inertia_Less = Lt_pu*wn_Inertia_Less^2/wb;
      |     Kp_Inertia_Less = 2*zeta_Inertia_Less*wn_Inertia_Less*Lt_pu/wb;
      |     
      |     % With Inertia
      |     Kc = 1/(Lt_pu);
      |     kp_GFo = zeta_GFo*sqrt(2/(H_GFo*wb*Kc));
      |     kd = 2*H_GFo*kp_GFo*Kc*wb;
      | 
      | % Virtual Impedance tuning
      |     X_VI = roots([1/DX_DR^2+1 2*Lt_pu Lt_pu^2-1/I_max_VI_pu^2]);
      |     X_VI = max(X_VI);
      |     Kp_Rvi_pu = X_VI/(DX_DR*(I_max_VI_pu-1)); 
      |     
      | % Set the chosen strategy
      |     if (gainpopup == 1)
      |         Chosen_Strategy = 1;
      |     elseif (gainpopup == 2)
      |         if (Param_Inertia == 1)
      |             Chosen_Strategy = 2;
      |         elseif (Param_Inertia == 2)
      |             Chosen_Strategy = 3;
      |         end
      |     end
      |     
      | % Set the frequency droop gain
      |     R = R_percent / 100;
      | 
      | % Compute the delay compensation between control and power parts
      |     if (Time_Step == -1)
      |         Solver_Time_Step = 0;
      |     else
      |         Solver_Time_Step = Time_Step;
      |     end
      | 
      | % Compute Initial Voltage of VSC 
      | %   from steady-state output transformer model and Loadflow result
      |     
      |     %Initialize correctly the LoadFlow bus parameters connected to PCC
      |     VLF = V0;
      |     ThetaLF = Theta0;
      |     %if (LFpopup == 'PQ')
      |     %    VLF = 1;
      |     %    ThetaLF = 0;
      |     %elseif (LFpopup == 'PV')
      |     %%    VLF = V0;
      |     %    ThetaLF = 0;        
      |     %end
      |     %set_param([gcb '/Load Flow Bus'],'Vref',num2str(VLF),'Vangle',num2str(ThetaLF));
      |     
      |     R1_pu = Rt_pu/2;
      |     L1_pu = Lt_pu/2;
      |     R2_pu = Rt_pu/2;
      |     L2_pu = Lt_pu/2;
      |     X1_pu = L1_pu;
      |     X2_pu = L2_pu;
      |     Xm_pu = Lm_pu;
      |     
      |     Zm_pu = 1/(1/Rm_pu+1/(1i*Xm_pu));
      | 
      |     S0=P0+1i*Q0;
      |     I2 = conj(S0)/(V0);
      | 
      |     Vm = (R2_pu+1i*X2_pu)*I2 + V0;
      |     Im = Vm/Zm_pu;
      | 
      |     I1 = I2 + Im;
      |     V1 = (R1_pu+1i*X1_pu) * I1 + Vm;
      | 
      |     Vvsc0 = abs(V1);
      |     Theta_vsc0 = angle(V1) * 180/pi+Theta0;
      |     
      |     Va0 = Vvsc0*sqrt(2)*Vb1*sin(Theta_vsc0*pi/180);
      |     Vb0 = Vvsc0*sqrt(2)*Vb1*sin(Theta_vsc0*pi/180-2*pi/3);
      |     Vc0 = Vvsc0*sqrt(2)*Vb1*sin(Theta_vsc0*pi/180+2*pi/3);
      |     
      | % Generate string to display LF results on Mask
      |     %str_tmp = fprintf("Vvsc0 = %d, Theta_vsc0 = %d°",Vvsc0,Theta_vsc0);
      |     mo = get_param(gcb,'MaskObject');
      |     mo.getDialogControl('LF_vsc_str').Prompt = ['V0 = ', num2str(Vvsc0),' pu, Angle = ', num2str(Theta_vsc0),'°'];
      |     mo.getDialogControl('LF_pcc_str').Prompt = ['V0 = ', num2str(V0),' pu, Angle = ', num2str(Theta0),'°'];
      |     mo.getDialogControl('LF_pcc_Power_str').Prompt = ['P0 = ', num2str(P0),' pu, Q0 = ', num2str(Q0),' pu'];
      |     %set_param([gcb],'LF_str',str_tmp);
      settings: OpenFcn=|
      | NameStr = get_param(gcb,'Name');
      | open_system(gcbh, 'Mask');
      | 
      | h2AllOpenDlgs = DAStudio.ToolRoot.getOpenDialogs;
      | 
      | for i=1:length(h2AllOpenDlgs)
      |     try
      |          %disp(h2AllOpenDlgs(i).getSource.getBlock.Name);
      |         Dialog_block_name = h2AllOpenDlgs(i).getSource.getBlock.Name;
      |          %strcmp(Dialog_block_name, NameStr),
      |         if (strcmp(h2AllOpenDlgs(i).getSource.getBlock.Name, NameStr))
      |             iPos = h2AllOpenDlgs(i).position;
      |             h2AllOpenDlgs(i).position = [iPos(1)   iPos(2)   iPos(3)*1.4   iPos(4)];
      |         end
      |     end
      | end
      mask Callback Advanced:
      | % Get the mask parameter values. This is a cell
      | %   array of character vectors.
      | maskStr = get_param(gcb,'Advanced');
      | p=Simulink.Mask.get(gcb);
      | 
      | % The pop-up menu is the first mask parameter.
      | %   Check the value selected in the pop-up
      | if strcmp(maskStr,'on'),
      | 
      |     % Set the visibility of both parameters on when
      |     %   User-defined is selected in the pop-up.
      |     p.getDialogControl('TVR').Visible='on';
      |     p.getDialogControl('TVI').Visible='on';
      |     %p.getDialogControl('LC_Filter').Visible='on';
      |     p.getDialogControl('Current_Sat').Visible='on';
      |     %p.getDialogControl('Param_Strat_3').Visible='off';
      | 
      | 
      | else
      | 
      |     % Set the visibility of both parameters on when
      |     %   User-defined is selected in the pop-up.
      |     p.getDialogControl('TVR').Visible='off';
      |     p.getDialogControl('TVI').Visible='off';
      |     %p.getDialogControl('LC_Filter').Visible='off';
      |     p.getDialogControl('Current_Sat').Visible='off';
      |     %p.getDialogControl('Param_Strat_3').Visible='off';
      | 
      | end
      mask TypeOptions gainpopup: Inertia Less | With Inertia
      mask Callback gainpopup:
      | % Get the mask parameter values. This is a cell
      | %   array of character vectors.
      | maskStr = get_param(gcb,'gainpopup');
      | p=Simulink.Mask.get(gcb);
      | 
      | % The pop-up menu is the first mask parameter.
      | %   Check the value selected in the pop-up
      | if strcmp(maskStr,'Inertia Less'),
      | 
      |     % Set the visibility of both parameters on when
      |     %   User-defined is selected in the pop-up.
      |     p.getDialogControl('No_Inertia').Visible='on';
      |     p.getDialogControl('Inertia').Visible='off';
      |     %p.getDialogControl('Param_Strat_3').Visible='off';
      | 
      | 
      | elseif strcmp(maskStr,'With Inertia'),
      | 
      |     % Set the visibility of both parameters on when
      |     %   User-defined is selected in the pop-up.
      |     p.getDialogControl('No_Inertia').Visible='off';
      |     p.getDialogControl('Inertia').Visible='on';
      |     %p.getDialogControl('Param_Strat_3').Visible='off';
      | 
      | 
      |     % Turn off the visibility of the Value field
      |     %   when User-defined is not selected.
      | 
      | else
      | 
      |     % Set the visibility of both parameters on when
      |     %   User-defined is selected in the pop-up.
      |     p.getDialogControl('No_Inertia').Visible='off';
      |     p.getDialogControl('Inertia').Visible='off';
      |     %p.getDialogControl('Param_Strat_3').Visible='off';
      | 
      | end
      mask TypeOptions Param_Inertia: VSM | PI
      mask TypeOptions LFpopup: Swing | PQ | PV
      mask Callback LFpopup:
      | % Get the mask parameter values. This is a cell
      | %   array of character vectors.
      | maskStr = get_param(gcb,'LFpopup');
      | p=Simulink.Mask.get(gcb);
      | 
      | % The pop-up menu is the first mask parameter.
      | %   Check the value selected in the pop-up
      | if strcmp(maskStr,'Swing'),
      | 
      |     % Set the visibility of both parameters on when
      |     %   User-defined is selected in the pop-up.
      |     p.getParameter('P0').Visible='off';
      |     p.getParameter('Q0').Visible='off';
      |     p.getParameter('V0').Visible='on';
      |     p.getParameter('Theta0').Visible='on';
      |     set_param([gcb '/Source_For_LF'],'BusType','swing');
      | 
      | elseif strcmp(maskStr,'PQ'),
      | 
      |     % Set the visibility of both parameters on when
      |     %   User-defined is selected in the pop-up.
      |     p.getParameter('P0').Visible='on';
      |     p.getParameter('Q0').Visible='on';
      |     p.getParameter('V0').Visible='off';
      |     p.getParameter('Theta0').Visible='off';
      |     set_param([gcb '/Source_For_LF'],'BusType','PQ');
      | 
      |     % Turn off the visibility of the Value field
      |     %   when User-defined is not selected.
      | else
      | 
      |     % Set the visibility of both parameters on when
      |     %   User-defined is selected in the pop-up.
      |     p.getParameter('P0').Visible='on';
      |     p.getParameter('Q0').Visible='off';
      |     p.getParameter('V0').Visible='on';
      |     p.getParameter('Theta0').Visible='off';
      |     set_param([gcb '/Source_For_LF'],'BusType','PV');
      | 
      | end
      mask DialogControl Nominal_Param Prompt: Nominal Value
      mask DialogControl Container20 Prompt: Passive Components
      mask DialogControl Control_Param Prompt: Control Parameter
      mask DialogControl Container13 Prompt: PLL
      mask DialogControl Container14 Prompt: Frequency Support
      mask DialogControl TVR Prompt: Transient Virtual Resistor
      mask DialogControl TVI Prompt: Virtual Impedance
      mask DialogControl Current_Sat Prompt: Current Limitation
      mask DialogControl Container18 Prompt: Control Strategy
      mask DialogControl LF_Param Prompt: Loadflow
      mask DialogControl Control4 Prompt: Initial Operating Point
      mask DialogControl Container24 Prompt: VSC side
      mask DialogControl LF_vsc_str Prompt: V0 = 1.0038 pu, Angle = 3.3244°
      mask DialogControl Container25 Prompt: PCC
      mask DialogControl LF_pcc_str Prompt: V0 = 1.0009 pu, Angle = 0.57242°
      mask DialogControl LF_pcc_Power_str Prompt: P0 = 0.2 pu, Q0 = 4.3368e-19 pu
      mask DialogControl UpdateLoadflow Prompt: Update Loadflow
      mask DialogControl UpdateLoadflow Callback: LoadFlow_VSC
      mask Display:
      | x1=0.05;
      | y1=0.2;
      | %
      | plot([0.5 0.5]+x1,[0.97,0.8]-y1)
      | plot([0.5 0.32]+x1,[0.80 0.71]-y1)
      | plot([0.32 0.32]+x1,[0.80 0.52]-y1)
      | plot([0.32 0.5]+x1,[0.62 0.52]-y1)
      | plot([0.5 0.5]+x1,[0.52 0.35]-y1)
      | plot([0.45 0.5 0.43]+x1,[0.59 0.52 0.51]-y1)
      | %
      | plot([0.28 0.28]+x1,[0.74 0.58]-y1)
      | plot([0.28 0.20]+x1,[0.66 0.66]-y1)
      | %
      | plot([0.5 0.63]+x1,[0.84 0.84]-y1)
      | plot([0.63 0.63]+x1,[0.84 0.72]-y1)
      | plot([0.63 0.59]+x1,[0.72 0.65]-y1)
      | plot([0.63 0.67]+x1,[0.72 0.65]-y1)
      | plot([0.59 0.67]+x1,[0.65 0.65]-y1)
      | plot([0.63 0.63]+x1,[0.65 0.47]-y1)
      | plot([0.5 0.63]+x1,[0.47 0.47]-y1)
      | plot([0.58 0.67]+x1,[0.72 0.72]-y1)
      | %
      | color('blue')
      | text(0.3,0.10,'L-Filter GFo')
      | port_label('input',1,'dE_set (pu)');
      | port_label('input',2,'dP_set (pu)');
      | port_label('output',1,'m');
      | port_label('rconn',1,'A');
      | port_label('rconn',2,'B');
      | port_label('rconn',3,'C');
  Scope : Scope  NumInputPorts=3
  Scope1 : Scope  NumInputPorts=3
  Step : Step  After=0.4  SampleTime=0
  Step1 : Step  After=0.4  SampleTime=0
  Step2 : Step  After=0.4  SampleTime=0
  Subsystem2 : Subsystem
      settings: OpenFcn=LoadFlow_VSC
      mask Display: color('blue'),disp('Update Loadflow')
  Three-Phase Series RLC Branch1 : spsThreePhaseSeriesRLCBranchLib/Three-Phase Series RLC Branch  LConnTagsString=A|B|C  RConnTagsString=A|B|C  BranchType=RL  Resistance=GRD00_Rg  Inductance=GRD00_Lg  Capacitance=1e-6  Measurements=None
  Three-Phase Series RLC Branch2 : spsThreePhaseSeriesRLCBranchLib/Three-Phase Series RLC Branch  LConnTagsString=A|B|C  RConnTagsString=A|B|C  BranchType=RL  Resistance=GRD00_Rg  Inductance=GRD00_Lg  Capacitance=1e-6  Measurements=None
  Three-Phase Series RLC Branch3 : spsThreePhaseSeriesRLCBranchLib/Three-Phase Series RLC Branch  LConnTagsString=A|B|C  RConnTagsString=A|B|C  BranchType=RL  Resistance=GRD00_Rg  Inductance=GRD00_Lg  Capacitance=1e-6  Measurements=None
  Three-Phase Source : spsThreePhaseSourceLib/Three-Phase Source  InternalConnection=Yg  VoltagePhases=off  Voltage=(400000)*1  PhaseAngle=0  Voltage_phases=[25e3 25e3 25e3]/sqrt(3)  PhaseAngles_phases=[0 -120 +120]  Frequency=50  NonIdealSource=off  SpecifyImpedance=off  Resistance=0.8929  Inductance=16.58e-3  ShortCircuitLevel=100e6  BaseVoltage=25e3  XRratio=7  BusType=swing  Pref=10e3  Qref=0  Prefabc=[10e3, 10e3, 10e3]  Qrefabc=[0, 0, 0]  Qmin=-inf  Qmax=inf
  powergui : spspowerguiLib/powergui  Priority=1  SimulationMode=Discrete  SampleTime=Time_Step  frequency=60  Iterations=50  frequencyindice=50  Pbase=1000000000  ErrMax=1e-6  UnitsV=kV  UnitsW=MW  buscounter=0  FunctionMessages=off  echomessages=off  EnableUseOfTLC=off  CurrentSourceSwitches=off  DisableSnubberDevices=off  DisableRonSwitches=off  DisableVfSwitches=off  DisplayEquations=off  AutomaticDiscreteSolvers=off  SolverType=Tustin/Backward Euler (TBE)  Interpol=off  ExternalGateDelay=off  methode=off  Ts=100  x0status=blocks  SPID=on  SwTol=0  HookPort=off  NonlinearTolerance=1e-4  nMaxIteration=100  ContinueOnMaxIteration=off  RestoreLinks=warning  ResistiveCurrentMeasurement=off  Frange=[0:2:500]  Ylog=off  Xlog=on  ShowGrid=off  save=off  variable=ZData  structure=0  ZoomFFT=off  StartTime=0.0  cycles=1  DisplayStyle=1  fundamental=60  FreqAxis=off  MaxFrequency=1000  frequencyindicesteady=1  RmsSteady=1  display=off
  wires:
  Energy Based/1(m) -> Bus Selector1/1
  Bus Selector1/1 -> [P_EB]  "<P>"
  Step/1 -> Energy Based/2(dP_set (pu))
  Step1/1 -> CCSC/2(dP_set (pu))
  Step2/1 -> Mean Model 2-Level L-filter/2(dP_set (pu))
  CCSC/1(m) -> Bus Selector2/1
  Mean Model 2-Level L-filter/1(m) -> Bus Selector3/1
  Bus to Vector/1 -> Scope/3  "P_VSC"
  Bus to Vector1/1 -> Scope/2  "P_CCSC"
  Bus to Vector2/1 -> Scope/1  "P_EB"
  Bus Selector1/2 -> [vm_dq_EB]  "<vm_dq>"
  Bus Selector2/1 -> [P_CCSC]  "<P>"
  Bus Selector2/2 -> [vm_dq_CCSC]  "<vm_dq>"
  Bus Selector3/1 -> [P_VSC]  "<P>"
  Bus Selector3/2 -> [vm_dq_VSC]  "<vm_dq>"
  [P_EB] -> Bus to Vector2/1
  [P_CCSC] -> Bus to Vector1/1
  [P_VSC] -> Bus to Vector/1
  Bus to Vector4/1 -> Scope1/2  "vm_CCSC"
  Bus to Vector5/1 -> Scope1/1  "vm_EB"
  Bus to Vector3/1 -> Scope1/3  "vm_VSC"
  [vm_dq_VSC] -> Bus to Vector3/1
  [vm_dq_CCSC] -> Bus to Vector4/1
  [vm_dq_EB] -> Bus to Vector5/1
  connections:
  Energy Based/RConn1 -- Three-Phase Series RLC Branch1/LConn1 -- Load Flow Bus/LConn1
  Three-Phase Series RLC Branch1/LConn2 -- Energy Based/RConn2
  Energy Based/RConn3 -- Three-Phase Series RLC Branch1/LConn3
  Three-Phase Series RLC Branch2/RConn1 -- Three-Phase Series RLC Branch3/RConn1 -- Three-Phase Source/RConn1 -- Load Flow Bus3/LConn1 -- Three-Phase Series RLC Branch1/RConn1
  Three-Phase Series RLC Branch2/RConn3 -- Three-Phase Series RLC Branch3/RConn3 -- Three-Phase Source/RConn3 -- Three-Phase Series RLC Branch1/RConn3
  Three-Phase Series RLC Branch2/RConn2 -- Three-Phase Series RLC Branch3/RConn2 -- Three-Phase Source/RConn2 -- Three-Phase Series RLC Branch1/RConn2
  CCSC/RConn3 -- Three-Phase Series RLC Branch2/LConn3
  CCSC/RConn2 -- Three-Phase Series RLC Branch2/LConn2
  Three-Phase Series RLC Branch2/LConn1 -- CCSC/RConn1 -- Load Flow Bus1/LConn1
  Mean Model 2-Level L-filter/RConn2 -- Three-Phase Series RLC Branch3/LConn2
  Load Flow Bus2/LConn1 -- Three-Phase Series RLC Branch3/LConn1 -- Mean Model 2-Level L-filter/RConn1
  Mean Model 2-Level L-filter/RConn3 -- Three-Phase Series RLC Branch3/LConn3
